simulink model "sfcndemo_port_constant"  (Simulink 6.0)
settings: Solver=FixedStepDiscrete  StartTime=0.0  StopTime=10  RelTol=1e-3
settings Model: Creator=The MathWorks Inc.  LastModifiedBy=batserve  ExtModeAutoUpdateStatusClock=off
settings OptimizationCC: BooleanDataType=off  InlineParams=on
settings DebuggingCC: CheckExecutionContextPreStartOutputMsg=on  CheckExecutionContextRuntimeOutputMsg=on  SolverPrmCheckMsg=none
settings HardwareCC: TargetUnknown=on

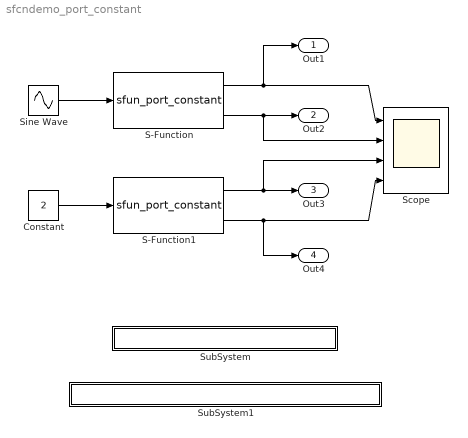
== system sfcndemo_port_constant ==
  Constant : Constant  Value=2
  S-Function : S-Function  FunctionName=sfun_port_constant  Parameters=5
  S-Function1 : S-Function  FunctionName=sfun_port_constant  Parameters=7
  Scope : Scope  NumInputPorts=4
      settings: TimeRange=10  YMin=-5~4~13~6  YMax=5~6~15~8
  Sine Wave : Sin  SampleTime=0
  SubSystem : Subsystem  PropExecContextAcrossSSBoundary=on
      settings: OpenFcn=edit(fullfile(matlabroot,'simulink','src','sfun_port_constant.c'))
      mask Display: disp('matlabroot\simulink\src\sfun_port_constant.c');
  SubSystem1 : Subsystem  PropExecContextAcrossSSBoundary=on
      settings: OpenFcn=edit(fullfile(matlabroot,'toolbox','simulink','blocks','tlc_c','sfun_port_constant.tlc'))
      mask Display: disp('matlabroot\toolbox\simulink\blocks\tlc_c\sfun_port_constant.tlc');
  Out1 : Outport
  Out2 : Outport  Port=2
  Out3 : Outport  Port=3
  Out4 : Outport  Port=4
  wires:
  Sine Wave/1 -> S-Function/1
  S-Function/1 -> Out1/1, Scope/1
  S-Function/2 -> Out2/1, Scope/2
  Constant/1 -> S-Function1/1
  S-Function1/1 -> Out3/1, Scope/3
  S-Function1/2 -> Scope/4, Out4/1

== system sfcndemo_port_constant/SubSystem ==

== system sfcndemo_port_constant/SubSystem1 ==
